simulink model "example_QProblemB"  (Simulink 7.4)
settings: Solver=VariableStepDiscrete  StartTime=0.0  StopTime=0.5  RelTol=1e-3
settings Model: Creator=jferreau  LastModifiedBy=chjofer2  ExtModeAutoUpdateStatusClock=off
settings OptimizationCC: InitFltsAndDblsToZero=on
settings DebuggingCC: SaveWithParameterizedLinksMsg=none  SignalResolutionControl=TryResolveAllWithWarning
settings GRTTargetCC: TargetFcnLib=ansi_tfl_tmw.mat

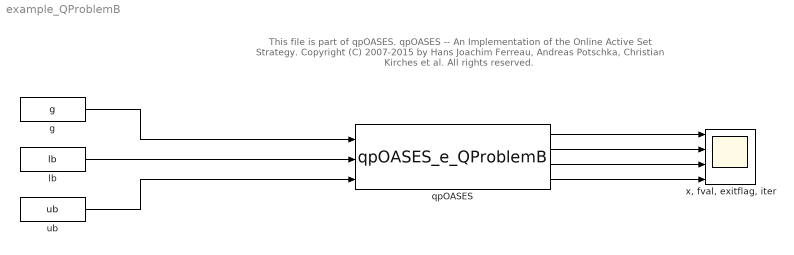
== system example_QProblemB ==
  note: This file is part of qpOASES.
      |
      | qpOASES -- An Implementation of the Online Active Set Strategy.
      | Copyright (C) 2007-2015 by Hans Joachim Ferreau, Andreas Potschka, Christian Kirches et al.
      | All rights reserved.
  g : FromWorkspace  VariableName=g  SampleTime=0.1  OutputAfterFinalValue=Holding final value
  lb : FromWorkspace  VariableName=lb  SampleTime=0.1  OutputAfterFinalValue=Holding final value
  qpOASES : S-Function  FunctionName=qpOASES_e_QProblemB  Parameters=H  EnableBusSupport=off
  ub : FromWorkspace  VariableName=ub  SampleTime=0.1  OutputAfterFinalValue=Holding final value
  "x, fval, exitflag, iter" : Scope  NumInputPorts=4
      settings: YMin=-5~-5~-5~-5  YMax=5~5~5~5
  wires:
  qpOASES/1 -> "x, fval, exitflag, iter"/1
  qpOASES/2 -> "x, fval, exitflag, iter"/2
  qpOASES/3 -> "x, fval, exitflag, iter"/3
  qpOASES/4 -> "x, fval, exitflag, iter"/4
  g/1 -> qpOASES/1
  lb/1 -> qpOASES/2
  ub/1 -> qpOASES/3
